simulink subsystem "sensorsonar"  (R2023b)
settings: Solver=VariableStepAuto  StartTime=0.0  StopTime=10.0  RelTol=1e-3
libraries: arduinolib x2
settings Model: Creator=Usuario_UMA  LastModifiedBy=Usuario_UMA

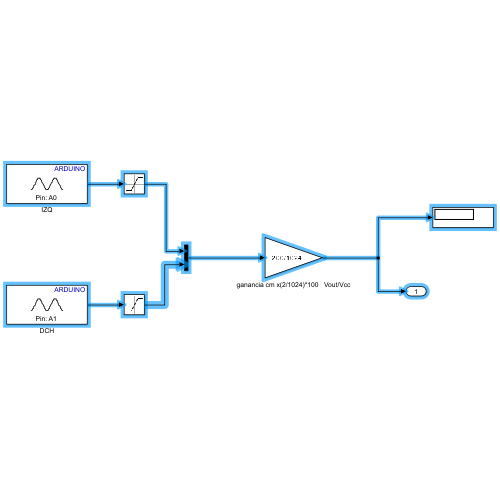
[thumbnail: Simulink's stored preview of the top-level diagram]
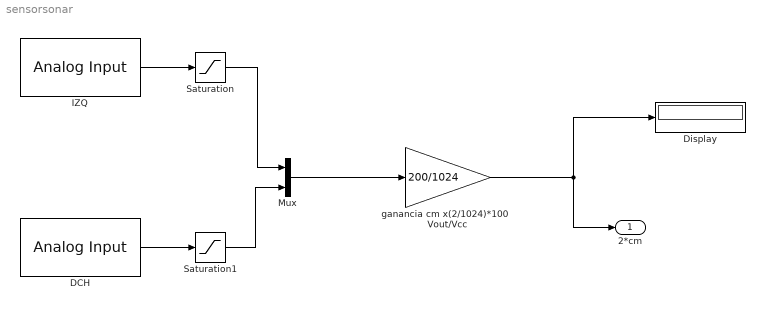
== system sensorsonar ==
  DCH : arduinolib/Analog Input  pinNumber=1  ReadResultsOnly=off  ConversionTriggerSource=Software  ExternalTriggerType=uint32( 0 )  OutputDataType=uint16  EnableConversionCompleteNotify=off  EnableOuputStatus=off  SampleTime=-1  blockPlatform=arduino
  Display : Display
  IZQ : arduinolib/Analog Input  pinNumber=0  ReadResultsOnly=off  ConversionTriggerSource=Software  ExternalTriggerType=uint32( 0 )  OutputDataType=uint16  EnableConversionCompleteNotify=off  EnableOuputStatus=off  SampleTime=-1  blockPlatform=arduino
  Mux : Mux  Inputs=2
  Saturation : Saturate
  Saturation1 : Saturate
  ganancia cm x(2/1024)*100   Vout/Vcc : Gain  Gain=200/1024
  2*cm : Outport
  wires:
  ganancia cm x(2/1024)*100   Vout/Vcc/1 -> 2*cm/1, Display/1
  Mux/1 -> ganancia cm x(2/1024)*100   Vout/Vcc/1
  Saturation/1 -> Mux/1
  IZQ/1 -> Saturation/1
  DCH/1 -> Saturation1/1
  Saturation1/1 -> Mux/2
